simulink model "NavV1_0421_2021a"  (R2021a)
settings: Solver=FixedStepAuto  StartTime=0.0  StopTime=589  FixedStep=dt  RelTol=1e-3
values from neighbouring files (symbols this model uses):
  dt = 0.01    [initNavigation.m]
  g0 = 9.798    [initNavigation.m]
  GPSdt = 0.1    [initNavigation.m]
undefined symbols (not defined in the file or in its folder): DiscIntNeverNeededParam, magnitude, param
libraries: simulink x14, simulink_extras x11, sharedtransform x7, dspstat3 x4, aerolibtransform2 x2, dspsolvers x2, aerolibconvert2 x1
(part 3 of 3)

== matlab function NavV1_0421_2021a/Sensor_Data_Process/Magn_Data_Process/gyro_preprocessing/MATLAB Function2 ==
  data: curr_input input single; curr_output output single; sample_freq input single; cutoff_freq input single
function curr_output = second_LPF_Butter_x(curr_input,sample_freq,cutoff_freq)
   persistent input_x;
   persistent output_x;

   if isempty(input_x)
       input_x = [0;0;0];
   end
   
   if isempty(output_x)
       output_x = [0;0;0];
   end
    B = [0,0,0];
    A = [0,0,0];
    M_PI_F = 3.1415926;
	fr = sample_freq / cutoff_freq;
	ohm = tan( M_PI_F / fr );
	c = 1.0 + 2.0 * cos( M_PI_F / 4.0 ) * ohm + ohm * ohm;
	B(1) = ohm * ohm / c;
	B(2) = 2.0 * B(1);
	B(3) = B(1);
	A(1) = 2.0 * ( ohm * ohm - 1.0) / c;
	A(2) = (1.0 - 2.0 * cos( M_PI_F / 4.0 ) * ohm + ohm * ohm) / c;
	%/*获取最新输入*/
	input_x(3) = curr_input;
	%/* Butterworth */
	output_x(3) =B(1) * input_x(3) + B(2) * input_x(2) +B(3) * input_x(1) - A(1) * output_x(2) - A(2) * output_x(1);
	curr_output = single(output_x(3));
   % /* 输入序列保存 */
	input_x(1) = input_x(2);
	input_x(2) = input_x(3);
	%/*输出序列保存 */
	output_x(1) = output_x(2);
	output_x(2) = output_x(3);
